simulink model "AA1111"  (R2018b)
settings: Solver=ode3  StartTime=0.0  StopTime=6000  FixedStep=T  RelTol=1e-3
PreLoadFcn:
  | Initial_LZ04
InitFcn:
  | Initial_LZ04
values from neighbouring files (symbols this model uses):
  Abg_GyroA = [0 0 1;0 1 0;-1 0 0]    [Initial_LZ04.m]
  Abg_GyroB = angle2dcm(-pi*3/4,0,-58/180*pi,'ZYX')    [Initial_LZ04.m]
  Abm_MmA = [0 -1 0;1 0 0;0 0 1]    [Initial_LZ04.m]
  Abm_MmB = [0 -1 0;1 0 0;0 0 1]    [Initial_LZ04.m]
  Att0 = 1*[80 0 0]'*pi/180    [Initial_LZ04.m]
  FixErr_StA = [15;15;15]*0*Kg_FixErr_St    [Initial_LZ04.m]
  FixErr_StB = ([15;15;15]*0+[10800;0;0])*Kg_FixErr_St    [Initial_LZ04.m]
  Fw_Mode = FW_Block(8,1)    [Initial.m]    (also in Initial_LZ04.m = 2)
  Fw_tao = 0.3    [Initial_LZ04.m]
  FwHmax = 4    [Initial_LZ04.m]
  FwTmax = FwTmax0    (= 0.05)    [Initial_LZ04.m]
  H0 = 0*[2;-2;-2;0]    [Initial_LZ04.m]
  Ib0_0 = [117.6 -1.39e-1 -1.14;-1.39e-1 101.9 -8.37e-2;-1.14 -8.37e-2 109.0]    [Initial_LZ04.m]
  jw = 0.0064    [Initial_LZ04.m]
  Matrix_I0 = [sin(50/180*pi)*cos(45/180*pi) -sin(50/180*pi)*cos(45/180*pi) -sin(50/180*pi)*cos(45/180*pi) sin(50/180*pi)*cos(45/180*pi);           sin(50/180*pi)*sin(45/180*pi) sin(50/180*pi)*sin(45/180*pi) -sin(50/180*pi)*sin(45/180*pi) -sin(50/180*pi)*sin(45/180*pi);           cos(50/180*pi) cos(50/180*pi) cos(50/180*pi) cos(50/180*pi)]    [Initial_LZ04.m]
  MtInfluence = 0    [Initial_LZ04.m]
  mu = 3.9860044e14    (= 398600440000000)    [Initial_LZ04.m]    (also in ZZ_User_Att.m)
  Ngc1 = [0.01;-0.02;-0.03]*Kg_Drift_Gyro*1+0*[0.001;-0.001;-0.001]    [Initial_LZ04.m]
  Ngc2 = [-0.02;0.01;-0.03]*Kg_Drift_Gyro    [Initial_LZ04.m]
  NgwxA = 0.005/60*sqrt(1/T_ctrl)*3*Kg_Noise_Gyro    [Initial_LZ04.m]
  NgwxB = 0.02/60*sqrt(1/T_ctrl)*3*Kg_Noise_Gyro    [Initial_LZ04.m]
  Noise_Mm = 7e-5*Kg_Noise_Mm    (= 7e-05)    [Initial_LZ04.m]
  Noise_StA = [3;3;30]*Kg_Noise_St    [Initial_LZ04.m]
  Noise_StB = [3;3;30]*Kg_Noise_St    [Initial_LZ04.m]
  OpenLoop_Att = 0    [Initial_LZ04.m]
  OpenLoop_Obt = 0    [Initial_LZ04.m]
  Qbs_StAFix = quatmultiply(angle2quat(pi,0,0,'XYZ'),angle2quat(-40/180*pi,20/180*pi,0,'XYZ'))    [Initial_LZ04.m]
  Qbs_StBFix = quatmultiply(angle2quat(pi,0,0,'XYZ'),angle2quat(40/180*pi,20/180*pi,0,'XYZ'))    [Initial_LZ04.m]
  Re = 6371.14e+3    (= 6371140)    [Initial.m]    (also in Initial_LZ04.m; ZZ_SystemApp.m)
  StartTime = [Year Month Day Hour Min Sec]'    [Initial_LZ04.m]
  T = T_PID - MainI.*[a_f/180*pi;0;0]    [Att_Ctrl.m]    (also in Initial_LZ04.m = 0.125; ZZ_Att.m = Tc(Axis))
  T_ctrl = 0.25    [Initial_LZ04.m]
  vx0 = sqrt(mu/a/(1-e^2))*(-sin(f)*sp(1)+(e+cos(f))*sq(1))    [Initial_LZ04.m]
  vy0 = sqrt(mu/a/(1-e^2))*(-sin(f)*sp(2)+(e+cos(f))*sq(2))    [Initial_LZ04.m]
  vz0 = sqrt(mu/a/(1-e^2))*(-sin(f)*sp(3)+(e+cos(f))*sq(3))    [Initial_LZ04.m]
  W_bi0 = 1*[0;-w0;0]+0*[2;-2;2]*pi/180    [Initial_LZ04.m]
  x0 = r0*(cos(omg+f)*cos(OMG)-sin(omg+f)*cos(i)*sin(OMG))    [Initial_LZ04.m]
  y0 = r0*(cos(omg+f)*sin(OMG)+sin(omg+f)*cos(i)*cos(OMG))    [Initial_LZ04.m]
  z0 = r0*sin(omg+f)*sin(i)    [Initial_LZ04.m]
undefined symbols (not defined in the file or in its folder): DiscIntNeverNeededParam, omegawXa
libraries: sharedutil x26, aerolibutil x15, simulink x12, sharedtransform x9, dspinverses x3, aerolibobsolete x1, vrlib x1
(part 3 of 3)

== system AA1111/Others/Oribit motion model/Compute osculating elements/     1/If Action Subsystem2 ==
  u : Inport
  T : Inport  Port=2
  Action Port : ActionPort  ActionType=then
  Product : Product  Inputs=3  RndMeth=Zero
  Sum : Sum  Inputs=|++  SaturateOnIntegerOverflow=on
  uz1 : Constant  Value=pi  VectorParams1D=off
  uz2 : Constant  Value=1/(2*pi)  VectorParams1D=off
  Out1 : Outport
  wires:
  u/1 -> Sum/1
  uz1/1 -> Sum/2
  Sum/1 -> Product/1
  uz2/1 -> Product/2
  Product/1 -> Out1/1
  T/1 -> Product/3

== system AA1111/Others/Oribit motion model/Compute osculating elements/   1/If Action Subsystem ==
  In1 : Inport
  Action Port : ActionPort  ActionType=then
  Out1 : Outport
  wires:
  In1/1 -> Out1/1

== system AA1111/Others/Oribit motion model/Compute osculating elements/   1/If Action Subsystem1 ==
  In1 : Inport
  Action Port : ActionPort  ActionType=else
  Constant : Constant  Value=2*pi
  Sum : Sum  Inputs=|+-  SaturateOnIntegerOverflow=on
  Out1 : Outport
  wires:
  Sum/1 -> Out1/1
  In1/1 -> Sum/2
  Constant/1 -> Sum/1

== system AA1111/Satellite Software/DataAcquisition/GyroMeasurment/TurntableModel/GyroOnTurntable ==
  dfai(¡ã/s) : Inport
  angle(¡ã) : Inport  Port=2
  Constant : Constant  Value=0
  Constant1 : Constant
  Demux1 : Demux  Outputs=3
  Gain : Gain  Gain=pi/180
  Gain1 : Gain
  Gain2 : Gain  Gain=-1
  Mux : Mux  Inputs=9
  Product : Product
  Product1 : Product
  Product2 : Product  Multiplication=Matrix(*)
  Reshape : Reshape  OutputDimensionality=Customize  OutputDimensions=[3,3]
  Terminator : Terminator
  Trigonometric Function2 : Trigonometry
  Trigonometric Function3 : Trigonometry  Operator=cos
  Trigonometric Function4 : Trigonometry
  Trigonometric Function5 : Trigonometry  Operator=cos
  wbi(¡ã/s) : Outport
  wires:
  Gain1/1 -> Mux/3
  Trigonometric Function3/1 -> Product/1, Product1/1
  Demux1/1 -> Terminator/1
  angle(¡ã)/1 -> Gain/1
  dfai(¡ã/s)/1 -> Product2/2
  Gain2/1 -> Mux/2
  Product2/1 -> wbi(¡ã/s)/1
  Reshape/1 -> Product2/1
  Constant1/1 -> Mux/9
  Product/1 -> Mux/1
  Product1/1 -> Gain2/1
  Trigonometric Function4/1 -> Product1/2, Mux/4
  Demux1/3 -> Trigonometric Function4/1, Trigonometric Function5/1
  Trigonometric Function2/1 -> Gain1/1
  Constant/1 -> Mux/6, Mux/7, Mux/8
  Mux/1 -> Reshape/1
  Gain/1 -> Demux1/1
  Trigonometric Function5/1 -> Product/2, Mux/5
  Demux1/2 -> Trigonometric Function2/1, Trigonometric Function3/1

== system AA1111/Satellite Software/DataAcquisition/GyroMeasurment/TurntableModel/Turntable Model ==
  W(¡ã/s) : Inport
  Constant : Constant  Value=360
  Demux : Demux  Outputs=3
  Integrator : Integrator
  Integrator1 : Integrator
  Integrator2 : Integrator
  Math Function : Math  Operator=mod  SaturateOnIntegerOverflow=on
  Math Function1 : Math  Operator=mod  SaturateOnIntegerOverflow=on
  Math Function2 : Math  Operator=mod  SaturateOnIntegerOverflow=on
  Mux : Mux  Inputs=3
  Angle(¡ã) : Outport
  wires:
  W(¡ã/s)/1 -> Demux/1
  Demux/1 -> Integrator/1
  Demux/2 -> Integrator1/1
  Demux/3 -> Integrator2/1
  Integrator/1 -> Math Function/1
  Mux/1 -> Angle(¡ã)/1
  Math Function/1 -> Mux/1
  Integrator1/1 -> Math Function1/1
  Integrator2/1 -> Math Function2/1
  Math Function2/1 -> Mux/3
  Math Function1/1 -> Mux/2
  Constant/1 -> Math Function2/2, Math Function1/2, Math Function/2

== system AA1111/Satellite Software/DataAcquisition/GyroMeasurment/TurntableModel/TurntableRotateSpeedCal ==
  wbi(¡ã/s) : Inport
  angle(¡ã) : Inport  Port=2
  Manual Switch : ManualSwitch
  Manual Switch1 : ManualSwitch
  TurntableRotateSpeedCal : Subsystem
  d_Att : Subsystem
  d_Att1 : Subsystem
  dfai(¡ã/s) : Outport
  wires:
  wbi(¡ã/s)/1 -> TurntableRotateSpeedCal/1(wbi(¡ã/s)), d_Att/1(wbi), d_Att1/1(wbi)
  angle(¡ã)/1 -> TurntableRotateSpeedCal/2(angle(¡ã)), d_Att/2(Att(xyz)), d_Att1/2(Att(xyz))
  TurntableRotateSpeedCal/1(dfai(¡ã/s)) -> Manual Switch/1
  d_Att/1(d_Att(xyz)) -> Manual Switch/2
  Manual Switch/1 -> Manual Switch1/1
  d_Att1/1(d_Att(xyz)) -> Manual Switch1/2
  Manual Switch1/1 -> dfai(¡ã/s)/1

== system AA1111/Satellite Software/DataAcquisition/OrbitElement measure/R//VToOrbitElement/  ==
  note: 0<=OMG<=2pi
  Hi : Inport
  Fcn1 : Fcn  Expr=u(1)
  Fcn2 : Fcn  Expr=u(2)
  If : If  IfExpression=u1 < 0
  If Action Subsystem : Subsystem  TreatAsAtomicUnit=on
  If Action Subsystem1 : Subsystem  TreatAsAtomicUnit=on
  Merge : Merge
  Mux3 : Mux  Inputs=2
  tg(OMG)=Hxi/(-Hyi) : Fcn  Expr=atan2(u[1],-u[2])
  OMG : Outport
  wires:
  Fcn1/1 -> Mux3/1
  Fcn2/1 -> Mux3/2
  Mux3/1 -> tg(OMG)=Hxi/(-Hyi)/1
  tg(OMG)=Hxi/(-Hyi)/1 -> If/1, If Action Subsystem/1(In1), If Action Subsystem1/1(In1)
  If/1 -> If Action Subsystem/Action
  If/2 -> If Action Subsystem1/Action
  If Action Subsystem/1(Out1) -> Merge/1
  If Action Subsystem1/1(Out1) -> Merge/2
  Merge/1 -> OMG/1
  Hi/1 -> Fcn1/1, Fcn2/1

== system AA1111/Satellite Software/DataAcquisition/OrbitElement measure/R//VToOrbitElement/      ==
  H_xyz : Inport
  R_xyz : Inport  Port=2
  3x3 Cross Product : sharedutil/3x3 Cross Product  aMode=aMode
      settings: SourceProductBaseCode=AE
  Dot Product4 : DotProduct  InputSameDT=on  OutDataTypeStr=Inherit: Inherit via internal rule
  Fcn1 : Fcn  Expr=acos(u[2]/(u[1]*u[3]))
  Fcn3 : Fcn  Expr=sqrt(u[1]^2+u[2]^2+u[3]^2)
  Fcn4 : Fcn  Expr=u[3]
  Fcn5 : Fcn  Expr=sqrt(u[1]^2+u[2]^2+u[3]^2)
  If Action Subsystem2 : Subsystem  TreatAsAtomicUnit=on
  If Action Subsystem3 : Subsystem  TreatAsAtomicUnit=on
  If1 : If
  Merge1 : Merge
  Mux1 : Mux  Inputs=3
  uz : Constant  Value=[0;0;1]  VectorParams1D=off
  u : Outport
  wires:
  uz/1 -> 3x3 Cross Product/1
  H_xyz/1 -> 3x3 Cross Product/2
  3x3 Cross Product/1 -> Dot Product4/1, Fcn5/1
  R_xyz/1 -> Fcn3/1, Dot Product4/2, Fcn4/1
  Fcn3/1 -> Mux1/3
  Dot Product4/1 -> Mux1/2
  Mux1/1 -> Fcn1/1
  Fcn4/1 -> If1/1
  If1/1 -> If Action Subsystem2/Action
  Fcn1/1 -> If Action Subsystem2/1(In1), If Action Subsystem3/1(In1)
  If Action Subsystem2/1(Out1) -> Merge1/1
  If Action Subsystem3/1(Out1) -> Merge1/2
  Merge1/1 -> u/1
  Fcn5/1 -> Mux1/1
  If1/2 -> If Action Subsystem3/Action

== system AA1111/Satellite Software/DataAcquisition/OrbitElement measure/R//VToOrbitElement/     1 ==
  note: Orbit Period T
  u : Inport
  a : Inport  Port=2
  Fcn : Fcn  Expr=2*pi*sqrt(u(1)^3/mu)
  If Action Subsystem1 : Subsystem  TreatAsAtomicUnit=on
  If Action Subsystem2 : Subsystem  TreatAsAtomicUnit=on
  If1 : If  IfExpression=u1 <pi
  Merge1 : Merge
  OrbitClock : Outport
  wires:
  If1/2 -> If Action Subsystem1/Action
  Merge1/1 -> OrbitClock/1
  If Action Subsystem1/1(Out1) -> Merge1/2
  If Action Subsystem2/1(Out1) -> Merge1/1
  If1/1 -> If Action Subsystem2/Action
  u/1 -> If Action Subsystem2/1(u), If1/1, If Action Subsystem1/1(u)
  a/1 -> Fcn/1
  Fcn/1 -> If Action Subsystem2/2(T), If Action Subsystem1/2(T)

== system AA1111/Satellite Software/DataAcquisition/OrbitElement measure/R//VToOrbitElement/   1 ==
  note: 0<=omg<=2pi
  note: Éý½»µãÊ¸Á¿Óë½üµØµãÊ¸Á¿µÄ¼Ð½Ç
  note: ¹ìµÀ½ÚÏßÊ¸Á¿N
  H_xyz : Inport
  V_xyz : Inport  Port=2
  R_xyz : Inport  Port=3
  3x3 Cross Product : sharedutil/3x3 Cross Product  aMode=aMode
      settings: SourceProductBaseCode=AE
  3x3 Cross Product1 : sharedutil/3x3 Cross Product  aMode=aMode
      settings: SourceProductBaseCode=AE
  Divide : Product  Inputs=*/
  Dot Product3 : DotProduct  InputSameDT=on  OutDataTypeStr=Inherit: Inherit via internal rule
  Fcn : Fcn  Expr=acos(u[2]/(u[1]*u[3]))
  Fcn2 : Fcn  Expr=u[3]
  Fcn3 : Fcn  Expr=sqrt(u[1]^2+u[2]^2+u[3]^2)
  Fcn5 : Fcn  Expr=sqrt(u[1]^2+u[2]^2+u[3]^2)
  Fcn6 : Fcn  Expr=sqrt(u[1]^2+u[2]^2+u[3]^2)
  Gain1 : Gain  Gain=180/pi
  Gain3 : Gain  Gain=mu  SaturateOnIntegerOverflow=on  OutDataTypeStr=Inherit: Same as input  ParamDataTypeStr=Inherit: Same as input
  If : If  IfExpression=u1 >= 0
  If Action Subsystem : Subsystem  TreatAsAtomicUnit=on
  If Action Subsystem1 : Subsystem  TreatAsAtomicUnit=on
  Merge : Merge
  Mux : Mux  Inputs=3
  Sum : Sum  Inputs=|--  SaturateOnIntegerOverflow=on
  uz : Constant  Value=[0;0;1]  VectorParams1D=off
  w{,1..4} (5 alike) : Scope
  omg : Outport
  wires:
  H_xyz/1 -> 3x3 Cross Product/2, 3x3 Cross Product1/1
  If Action Subsystem1/1(Out1) -> Merge/2
  If Action Subsystem/1(Out1) -> Merge/1
  Fcn/1 -> If Action Subsystem1/1(In1), If Action Subsystem/1(In1), Gain1/1
  Fcn2/1 -> If/1, w1/1
  Mux/1 -> Fcn/1
  Fcn6/1 -> Mux/3, w4/1
  Sum/1 -> Fcn2/1, Dot Product3/2, Fcn6/1
  Divide/1 -> Sum/2, w2/1
  Fcn3/1 -> Divide/2
  3x3 Cross Product/1 -> Fcn5/1, Dot Product3/1
  uz/1 -> 3x3 Cross Product/1
  3x3 Cross Product1/1 -> Sum/1, w3/1
  R_xyz/1 -> Fcn3/1, Gain3/1
  Dot Product3/1 -> Mux/2
  V_xyz/1 -> 3x3 Cross Product1/2
  Merge/1 -> omg/1
  If/1 -> If Action Subsystem/Action
  If/2 -> If Action Subsystem1/Action
  Gain1/1 -> w/1
  Gain3/1 -> Divide/1
  Fcn5/1 -> Mux/1

== system AA1111/Satellite Software/DataAcquisition/OrbitElement measure/qip/2 ==
  q : Inport
  Demux : Demux
  Gain1 : Gain  Gain=-1  SaturateOnIntegerOverflow=on  OutDataTypeStr=Inherit: Same as input  ParamDataTypeStr=Inherit: Same as input
  Gain2 : Gain  Gain=-1  SaturateOnIntegerOverflow=on  OutDataTypeStr=Inherit: Same as input  ParamDataTypeStr=Inherit: Same as input
  Gain3 : Gain  Gain=-1  SaturateOnIntegerOverflow=on  OutDataTypeStr=Inherit: Same as input  ParamDataTypeStr=Inherit: Same as input
  Mux : Mux
  inv(q) : Outport
  wires:
  Gain3/1 -> Mux/4
  Demux/4 -> Gain3/1
  Demux/3 -> Gain2/1
  Demux/2 -> Gain1/1
  Demux/1 -> Mux/1
  Gain2/1 -> Mux/3
  Gain1/1 -> Mux/2
  Mux/1 -> inv(q)/1
  q/1 -> Demux/1

== system AA1111/Others/Attitude Kinematics Equations & Attitude Dynamics Equations/Kinetics/Qob 2 Qib/qip/2 ==
  q : Inport
  Demux : Demux
  Gain1 : Gain  Gain=-1  SaturateOnIntegerOverflow=on  OutDataTypeStr=Inherit: Same as input  ParamDataTypeStr=Inherit: Same as input
  Gain2 : Gain  Gain=-1  SaturateOnIntegerOverflow=on  OutDataTypeStr=Inherit: Same as input  ParamDataTypeStr=Inherit: Same as input
  Gain3 : Gain  Gain=-1  SaturateOnIntegerOverflow=on  OutDataTypeStr=Inherit: Same as input  ParamDataTypeStr=Inherit: Same as input
  Mux : Mux
  inv(q) : Outport
  wires:
  q/1 -> Demux/1
  Mux/1 -> inv(q)/1
  Gain1/1 -> Mux/2
  Gain2/1 -> Mux/3
  Demux/1 -> Mux/1
  Demux/2 -> Gain1/1
  Demux/3 -> Gain2/1
  Demux/4 -> Gain3/1
  Gain3/1 -> Mux/4

== system AA1111/Others/Attitude Kinematics Equations & Attitude Dynamics Equations/Kinetics/Qob 2 Qib1/qip/2 ==
  q : Inport
  Demux : Demux
  Gain1 : Gain  Gain=-1  SaturateOnIntegerOverflow=on  OutDataTypeStr=Inherit: Same as input  ParamDataTypeStr=Inherit: Same as input
  Gain2 : Gain  Gain=-1  SaturateOnIntegerOverflow=on  OutDataTypeStr=Inherit: Same as input  ParamDataTypeStr=Inherit: Same as input
  Gain3 : Gain  Gain=-1  SaturateOnIntegerOverflow=on  OutDataTypeStr=Inherit: Same as input  ParamDataTypeStr=Inherit: Same as input
  Mux : Mux
  inv(q) : Outport
  wires:
  Gain3/1 -> Mux/4
  Demux/4 -> Gain3/1
  Demux/3 -> Gain2/1
  Demux/2 -> Gain1/1
  Demux/1 -> Mux/1
  Gain2/1 -> Mux/3
  Gain1/1 -> Mux/2
  Mux/1 -> inv(q)/1
  q/1 -> Demux/1

== system AA1111/Others/Disturbing torque/Compute geomagnetism1/Subsystem/Subsystem1/-pi~pi ==
  In1 : Inport
  If Action Subsystem1 : Subsystem  TreatAsAtomicUnit=on
  If Action Subsystem2 : Subsystem  TreatAsAtomicUnit=on
  If Action Subsystem3 : Subsystem  TreatAsAtomicUnit=on
  If Action Subsystem4 : Subsystem  TreatAsAtomicUnit=on
  If1 : If  IfExpression=u1>pi
  If2 : If  IfExpression=u1<0
  Merge1 : Merge
  Merge2 : Merge
  Out1 : Outport
  wires:
  Merge2/1 -> If Action Subsystem3/1(In), If Action Subsystem4/1(In), If1/1
  If Action Subsystem2/1(Out) -> Merge2/2
  If Action Subsystem1/1(Out) -> Merge2/1
  If2/2 -> If Action Subsystem2/Action
  If2/1 -> If Action Subsystem1/Action
  In1/1 -> If Action Subsystem2/1(In), If Action Subsystem1/1(In), If2/1
  Merge1/1 -> Out1/1
  If1/1 -> If Action Subsystem4/Action
  If Action Subsystem4/1(Out) -> Merge1/1
  If1/2 -> If Action Subsystem3/Action
  If Action Subsystem3/1(Out) -> Merge1/2

== system AA1111/Others/Disturbing torque/Compute geomagnetism1/Subsystem/Subsystem1/-pi~pi1 ==
  In1 : Inport
  If Action Subsystem1 : Subsystem  TreatAsAtomicUnit=on
  If Action Subsystem2 : Subsystem  TreatAsAtomicUnit=on
  If Action Subsystem3 : Subsystem  TreatAsAtomicUnit=on
  If Action Subsystem4 : Subsystem  TreatAsAtomicUnit=on
  If1 : If  IfExpression=u1>pi
  If2 : If  IfExpression=u1<0
  Merge1 : Merge
  Merge2 : Merge
  Out1 : Outport
  wires:
  If Action Subsystem3/1(Out) -> Merge1/2
  If1/2 -> If Action Subsystem3/Action
  If Action Subsystem4/1(Out) -> Merge1/1
  If1/1 -> If Action Subsystem4/Action
  Merge1/1 -> Out1/1
  In1/1 -> If2/1, If Action Subsystem1/1(In), If Action Subsystem2/1(In)
  If2/1 -> If Action Subsystem1/Action
  If2/2 -> If Action Subsystem2/Action
  If Action Subsystem1/1(Out) -> Merge2/1
  If Action Subsystem2/1(Out) -> Merge2/2
  Merge2/1 -> If1/1, If Action Subsystem4/1(In), If Action Subsystem3/1(In)

== system AA1111/Others/Disturbing torque/Compute geomagnetism1/Subsystem/Subsystem1/If Action Subsystem1 ==
  In : Inport
  Action Port : ActionPort  ActionType=else
  Demux : Demux  Outputs=2
  If : If  NumInputs=2  IfExpression=u2>0
  If Action Subsystem1 : Subsystem  TreatAsAtomicUnit=on
  If Action Subsystem2 : Subsystem  TreatAsAtomicUnit=on
  Merge : Merge
  Out : Outport
  wires:
  If/1 -> If Action Subsystem1/Action
  In/1 -> Demux/1
  Demux/1 -> If/1
  Demux/2 -> If/2
  If/2 -> If Action Subsystem2/Action
  If Action Subsystem1/1(Out) -> Merge/1
  If Action Subsystem2/1(Out) -> Merge/2
  Merge/1 -> Out/1

== system AA1111/Others/Disturbing torque/Compute geomagnetism1/Subsystem/Subsystem1/If Action Subsystem2 ==
  In : Inport
  Action Port : ActionPort  ActionType=then
  Fcn4 : Fcn  Expr=atan2(u[2],u[1])
  Out : Outport
  wires:
  In/1 -> Fcn4/1
  Fcn4/1 -> Out/1

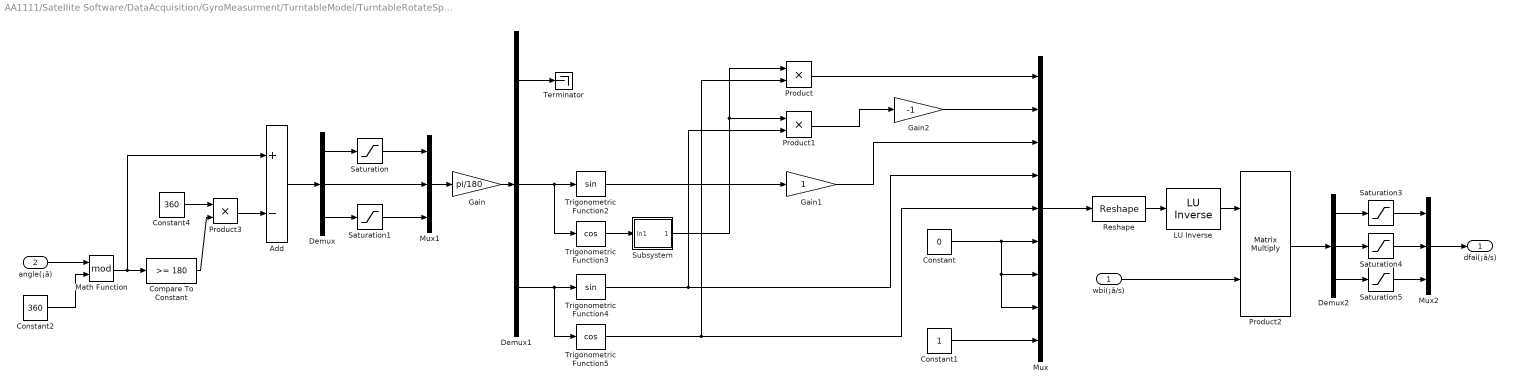
== system AA1111/Satellite Software/DataAcquisition/GyroMeasurment/TurntableModel/TurntableRotateSpeedCal/TurntableRotateSpeedCal ==
  wbi(¡ã/s) : Inport
  angle(¡ã) : Inport  Port=2
  " LU Inverse" : dspinverses/ LU Inverse
      settings: SourceProductName=DSP System Toolbox
  Add : Sum  Inputs=+-
  Compare To Constant : simulink/Logic and Bit Operations/Compare To Constant  relop=>=  const=180  OutDataTypeStr=uint8
  Constant : Constant  Value=0
  Constant1 : Constant
  Constant2 : Constant  Value=360
  Constant4 : Constant  Value=360
  Demux : Demux  Outputs=3
  Demux1 : Demux  Outputs=3
  Demux2 : Demux  Outputs=3
  Gain : Gain  Gain=pi/180
  Gain1 : Gain
  Gain2 : Gain  Gain=-1
  Math Function : Math  Operator=mod  SaturateOnIntegerOverflow=on
  Mux : Mux  Inputs=9
  Mux1 : Mux  Inputs=3
  Mux2 : Mux  Inputs=3
  Product : Product
  Product1 : Product
  Product2 : Product  Multiplication=Matrix(*)
  Product3 : Product
  Reshape : Reshape  OutputDimensionality=Customize  OutputDimensions=[3,3]
  Saturation : Saturate  UpperLimit=179  LowerLimit=-179
  Saturation1 : Saturate  UpperLimit=179  LowerLimit=-179
  Saturation3 : Saturate  UpperLimit=5  LowerLimit=-5
  Saturation4 : Saturate  UpperLimit=5  LowerLimit=-5
  Saturation5 : Saturate  UpperLimit=5  LowerLimit=-5
  Subsystem : Subsystem
  Terminator : Terminator
  Trigonometric Function2 : Trigonometry
  Trigonometric Function3 : Trigonometry  Operator=cos
  Trigonometric Function4 : Trigonometry
  Trigonometric Function5 : Trigonometry  Operator=cos
  dfai(¡ã/s) : Outport
  wires:
  Demux1/2 -> Trigonometric Function3/1, Trigonometric Function2/1
  Trigonometric Function5/1 -> Mux/5, Product/2
  Gain/1 -> Demux1/1
  Mux/1 -> Reshape/1
  Constant/1 -> Mux/6, Mux/7, Mux/8
  Trigonometric Function2/1 -> Gain1/1
  Demux1/3 -> Trigonometric Function5/1, Trigonometric Function4/1
  Trigonometric Function4/1 -> Product1/2, Mux/4
  Product1/1 -> Gain2/1
  Product/1 -> Mux/1
  Constant1/1 -> Mux/9
  " LU Inverse"/1 -> Product2/1
  Reshape/1 -> " LU Inverse"/1
  Math Function/1 -> Add/1, Compare To Constant/1
  Constant2/1 -> Math Function/2
  Constant4/1 -> Product3/1
  Compare To Constant/1 -> Product3/2
  Product3/1 -> Add/2
  Add/1 -> Demux/1
  Gain2/1 -> Mux/2
  Demux/2 -> Mux1/2
  Demux/3 -> Saturation1/1
  Saturation/1 -> Mux1/1
  Mux1/1 -> Gain/1
  Demux/1 -> Saturation/1
  Saturation1/1 -> Mux1/3
  wbi(¡ã/s)/1 -> Product2/2
  angle(¡ã)/1 -> Math Function/1
  Demux1/1 -> Terminator/1
  Subsystem/1(Out1) -> Product1/1, Product/1
  Trigonometric Function3/1 -> Subsystem/1(In1)
  Gain1/1 -> Mux/3
  Demux2/2 -> Saturation4/1
  Demux2/3 -> Saturation5/1
  Saturation3/1 -> Mux2/1
  Mux2/1 -> dfai(¡ã/s)/1
  Demux2/1 -> Saturation3/1
  Saturation5/1 -> Mux2/3
  Saturation4/1 -> Mux2/2
  Product2/1 -> Demux2/1

== system AA1111/Satellite Software/DataAcquisition/GyroMeasurment/TurntableModel/TurntableRotateSpeedCal/d_Att ==
  note: 0.0349 ¶ÔÓ¦88deg
      | 0.0872¶ÔÓ¦85deg
  wbi : Inport
  Att(xyz) : Inport  Port=2
  Demux2 : Demux  Outputs=3
  Fcn : Fcn  Expr=abs(cos(u(2)/180*pi))
  If : If  IfExpression=u1 <= 0.0349
  If Action Subsystem1 : Subsystem  TreatAsAtomicUnit=on
  If Action Subsystem2 : Subsystem  TreatAsAtomicUnit=on
  Integer Delay : Delay  DelayLength=1  InputProcessing=Inherited
  Merge : Merge
  Mux2 : Mux  Inputs=3
  Saturation3 : Saturate  UpperLimit=5  LowerLimit=-5
  Saturation4 : Saturate  UpperLimit=5  LowerLimit=-5
  Saturation5 : Saturate  UpperLimit=5  LowerLimit=-5
  d_Att(xyz) : Outport
  wires:
  If Action Subsystem2/1(Out2) -> Merge/1
  If/1 -> If Action Subsystem2/Action
  If Action Subsystem1/1(dfai(¡ã/s)) -> Merge/2
  If/2 -> If Action Subsystem1/Action
  Fcn/1 -> If/1
  Att(xyz)/1 -> If Action Subsystem1/2(angle(¡ã)), Fcn/1
  wbi/1 -> If Action Subsystem1/1(wbi(¡ã/s))
  Integer Delay/1 -> If Action Subsystem2/1(In2)
  Demux2/2 -> Saturation4/1
  Demux2/3 -> Saturation5/1
  Saturation3/1 -> Mux2/1
  Mux2/1 -> d_Att(xyz)/1, Integer Delay/1
  Demux2/1 -> Saturation3/1
  Saturation5/1 -> Mux2/3
  Saturation4/1 -> Mux2/2
  Merge/1 -> Demux2/1

== system AA1111/Satellite Software/DataAcquisition/GyroMeasurment/TurntableModel/TurntableRotateSpeedCal/d_Att1 ==
  wbi : Inport
  Att(xyz) : Inport  Port=2
  Demux2 : Demux  Outputs=3
  If Action Subsystem1 : Subsystem  TreatAsAtomicUnit=on
  Mux2 : Mux  Inputs=3
  Saturation3 : Saturate  UpperLimit=5  LowerLimit=-5
  Saturation4 : Saturate  UpperLimit=5  LowerLimit=-5
  Saturation5 : Saturate  UpperLimit=5  LowerLimit=-5
  d_Att(xyz) : Outport
  wires:
  Saturation4/1 -> Mux2/2
  Saturation5/1 -> Mux2/3
  Demux2/1 -> Saturation3/1
  Mux2/1 -> d_Att(xyz)/1
  Saturation3/1 -> Mux2/1
  Demux2/3 -> Saturation5/1
  Demux2/2 -> Saturation4/1
  wbi/1 -> If Action Subsystem1/1(wbi(¡ã/s))
  Att(xyz)/1 -> If Action Subsystem1/2(angle(¡ã))
  If Action Subsystem1/1(dfai(¡ã/s)) -> Demux2/1

== system AA1111/Satellite Software/DataAcquisition/OrbitElement measure/R//VToOrbitElement/ /If Action Subsystem ==
  note: In+2pi, due to OMG's Range=[0 2*pi],
      | and atan2's Range=[-pi pi]
  In1 : Inport
  Action Port : ActionPort  ActionType=then
  Constant : Constant  Value=2*pi
  Sum : Sum  Inputs=|++  SaturateOnIntegerOverflow=on
  Out1 : Outport
  wires:
  In1/1 -> Sum/1
  Sum/1 -> Out1/1
  Constant/1 -> Sum/2

== system AA1111/Satellite Software/DataAcquisition/OrbitElement measure/R//VToOrbitElement/ /If Action Subsystem1 ==
  In1 : Inport
  Action Port : ActionPort  ActionType=else
  Out1 : Outport
  wires:
  In1/1 -> Out1/1

== system AA1111/Satellite Software/DataAcquisition/OrbitElement measure/R//VToOrbitElement/     /If Action Subsystem2 ==
  In1 : Inport
  Action Port : ActionPort  ActionType=then
  Out1 : Outport
  wires:
  In1/1 -> Out1/1

== system AA1111/Satellite Software/DataAcquisition/OrbitElement measure/R//VToOrbitElement/     /If Action Subsystem3 ==
  In1 : Inport
  Action Port : ActionPort  ActionType=else
  Constant : Constant  Value=2*pi
  Sum : Sum  Inputs=|+-  SaturateOnIntegerOverflow=on
  Out1 : Outport
  wires:
  Sum/1 -> Out1/1
  In1/1 -> Sum/2
  Constant/1 -> Sum/1

== system AA1111/Satellite Software/DataAcquisition/OrbitElement measure/R//VToOrbitElement/     1/If Action Subsystem1 ==
  u : Inport
  T : Inport  Port=2
  Action Port : ActionPort  ActionType=else
  Product : Product  Inputs=3  RndMeth=Zero
  Sum : Sum  Inputs=|+-  SaturateOnIntegerOverflow=on
  uz1 : Constant  Value=pi  VectorParams1D=off
  uz2 : Constant  Value=1/(2*pi)  VectorParams1D=off
  Out1 : Outport
  wires:
  Product/1 -> Out1/1
  uz2/1 -> Product/2
  Sum/1 -> Product/1
  uz1/1 -> Sum/2
  u/1 -> Sum/1
  T/1 -> Product/3

== system AA1111/Satellite Software/DataAcquisition/OrbitElement measure/R//VToOrbitElement/     1/If Action Subsystem2 ==
  u : Inport
  T : Inport  Port=2
  Action Port : ActionPort  ActionType=then
  Product : Product  Inputs=3  RndMeth=Zero
  Sum : Sum  Inputs=|++  SaturateOnIntegerOverflow=on
  uz1 : Constant  Value=pi  VectorParams1D=off
  uz2 : Constant  Value=1/(2*pi)  VectorParams1D=off
  Out1 : Outport
  wires:
  u/1 -> Sum/1
  uz1/1 -> Sum/2
  Sum/1 -> Product/1
  uz2/1 -> Product/2
  Product/1 -> Out1/1
  T/1 -> Product/3

== system AA1111/Satellite Software/DataAcquisition/OrbitElement measure/R//VToOrbitElement/   1/If Action Subsystem ==
  In1 : Inport
  Action Port : ActionPort  ActionType=then
  Out1 : Outport
  wires:
  In1/1 -> Out1/1

== system AA1111/Satellite Software/DataAcquisition/OrbitElement measure/R//VToOrbitElement/   1/If Action Subsystem1 ==
  In1 : Inport
  Action Port : ActionPort  ActionType=else
  Constant : Constant  Value=2*pi
  Sum : Sum  Inputs=|+-  SaturateOnIntegerOverflow=on
  Out1 : Outport
  wires:
  Sum/1 -> Out1/1
  In1/1 -> Sum/2
  Constant/1 -> Sum/1

== system AA1111/Others/Disturbing torque/Compute geomagnetism1/Subsystem/Subsystem1/-pi~pi/If Action Subsystem1 ==
  In : Inport
  Action Port : ActionPort  ActionType=then
  Fcn4 : Fcn  Expr=u(1)+2*pi
  Out : Outport
  wires:
  In/1 -> Fcn4/1
  Fcn4/1 -> Out/1

== system AA1111/Others/Disturbing torque/Compute geomagnetism1/Subsystem/Subsystem1/-pi~pi/If Action Subsystem2 ==
  In : Inport
  Action Port : ActionPort  ActionType=else
  Out : Outport
  wires:
  In/1 -> Out/1

== system AA1111/Others/Disturbing torque/Compute geomagnetism1/Subsystem/Subsystem1/-pi~pi/If Action Subsystem3 ==
  In : Inport
  Action Port : ActionPort  ActionType=else
  Out : Outport
  wires:
  In/1 -> Out/1

== system AA1111/Others/Disturbing torque/Compute geomagnetism1/Subsystem/Subsystem1/-pi~pi/If Action Subsystem4 ==
  In : Inport
  Action Port : ActionPort  ActionType=then
  Fcn4 : Fcn  Expr=u(1)-2*pi
  Out : Outport
  wires:
  Fcn4/1 -> Out/1
  In/1 -> Fcn4/1

== system AA1111/Others/Disturbing torque/Compute geomagnetism1/Subsystem/Subsystem1/-pi~pi1/If Action Subsystem1 ==
  In : Inport
  Action Port : ActionPort  ActionType=then
  Fcn4 : Fcn  Expr=u(1)+2*pi
  Out : Outport
  wires:
  Fcn4/1 -> Out/1
  In/1 -> Fcn4/1

== system AA1111/Others/Disturbing torque/Compute geomagnetism1/Subsystem/Subsystem1/-pi~pi1/If Action Subsystem2 ==
  In : Inport
  Action Port : ActionPort  ActionType=else
  Out : Outport
  wires:
  In/1 -> Out/1

== system AA1111/Others/Disturbing torque/Compute geomagnetism1/Subsystem/Subsystem1/-pi~pi1/If Action Subsystem3 ==
  In : Inport
  Action Port : ActionPort  ActionType=else
  Out : Outport
  wires:
  In/1 -> Out/1

== system AA1111/Others/Disturbing torque/Compute geomagnetism1/Subsystem/Subsystem1/-pi~pi1/If Action Subsystem4 ==
  In : Inport
  Action Port : ActionPort  ActionType=then
  Fcn4 : Fcn  Expr=u(1)-2*pi
  Out : Outport
  wires:
  In/1 -> Fcn4/1
  Fcn4/1 -> Out/1

== system AA1111/Others/Disturbing torque/Compute geomagnetism1/Subsystem/Subsystem1/If Action Subsystem1/If Action Subsystem1 ==
  Action Port : ActionPort  ActionType=then
  Constant : Constant  Value=pi/2
  Out : Outport  InitialOutput=pi/2
  wires:
  Constant/1 -> Out/1

== system AA1111/Others/Disturbing torque/Compute geomagnetism1/Subsystem/Subsystem1/If Action Subsystem1/If Action Subsystem2 ==
  Action Port : ActionPort  ActionType=else
  Constant : Constant  Value=3*pi/2
  Out : Outport  InitialOutput=1.5*pi
  wires:
  Constant/1 -> Out/1

== system AA1111/Satellite Software/DataAcquisition/GyroMeasurment/TurntableModel/TurntableRotateSpeedCal/TurntableRotateSpeedCal/Subsystem ==
  In1 : Inport
  Abs1 : Abs
  Constant1 : Constant  Value=0.005
  Product1 : Product
  Sign : Signum
  Switch : Switch  Criteria=u2 > Threshold  Threshold=0.005
  Out1 : Outport
  wires:
  Abs1/1 -> Switch/2
  Sign/1 -> Product1/1
  Constant1/1 -> Product1/2
  Product1/1 -> Switch/3
  Switch/1 -> Out1/1
  In1/1 -> Switch/1, Abs1/1, Sign/1

== system AA1111/Satellite Software/DataAcquisition/GyroMeasurment/TurntableModel/TurntableRotateSpeedCal/d_Att/If Action Subsystem1 ==
  wbi(¡ã/s) : Inport
  angle(¡ã) : Inport  Port=2
  Action Port : ActionPort  ActionType=else
  " LU Inverse" : dspinverses/ LU Inverse
      settings: SourceProductName=DSP System Toolbox
  Constant : Constant  Value=0
  Constant1 : Constant
  Demux1 : Demux  Outputs=3
  Gain : Gain  Gain=pi/180
  Gain1 : Gain
  Gain2 : Gain  Gain=-1
  Mux : Mux  Inputs=9
  Product : Product
  Product1 : Product
  Product2 : Product  Multiplication=Matrix(*)
  Reshape : Reshape  OutputDimensionality=Customize  OutputDimensions=[3,3]
  Terminator : Terminator
  Trigonometric Function2 : Trigonometry
  Trigonometric Function3 : Trigonometry  Operator=cos
  Trigonometric Function4 : Trigonometry
  Trigonometric Function5 : Trigonometry  Operator=cos
  dfai(¡ã/s) : Outport
  wires:
  Gain1/1 -> Mux/3
  Trigonometric Function3/1 -> Product/1, Product1/1
  Demux1/1 -> Terminator/1
  angle(¡ã)/1 -> Gain/1
  wbi(¡ã/s)/1 -> Product2/2
  Gain2/1 -> Mux/2
  Product2/1 -> dfai(¡ã/s)/1
  Reshape/1 -> " LU Inverse"/1
  " LU Inverse"/1 -> Product2/1
  Constant1/1 -> Mux/9
  Product/1 -> Mux/1
  Product1/1 -> Gain2/1
  Trigonometric Function4/1 -> Product1/2, Mux/4
  Demux1/3 -> Trigonometric Function4/1, Trigonometric Function5/1
  Trigonometric Function2/1 -> Gain1/1
  Constant/1 -> Mux/6, Mux/7, Mux/8
  Mux/1 -> Reshape/1
  Gain/1 -> Demux1/1
  Trigonometric Function5/1 -> Product/2, Mux/5
  Demux1/2 -> Trigonometric Function2/1, Trigonometric Function3/1

== system AA1111/Satellite Software/DataAcquisition/GyroMeasurment/TurntableModel/TurntableRotateSpeedCal/d_Att/If Action Subsystem2 ==
  In2 : Inport
  Action Port : ActionPort  ActionType=then
  Out2 : Outport
  wires:
  In2/1 -> Out2/1

== system AA1111/Satellite Software/DataAcquisition/GyroMeasurment/TurntableModel/TurntableRotateSpeedCal/d_Att1/If Action Subsystem1 ==
  wbi(¡ã/s) : Inport
  angle(¡ã) : Inport  Port=2
  " LU Inverse" : dspinverses/ LU Inverse
      settings: SourceProductName=DSP System Toolbox
  Constant : Constant  Value=0
  Constant1 : Constant
  Demux1 : Demux  Outputs=3
  Gain : Gain  Gain=pi/180
  Gain1 : Gain
  Gain2 : Gain  Gain=-1
  Mux : Mux  Inputs=9
  Product : Product
  Product1 : Product
  Product2 : Product  Multiplication=Matrix(*)
  Reshape : Reshape  OutputDimensionality=Customize  OutputDimensions=[3,3]
  Terminator : Terminator
  Trigonometric Function2 : Trigonometry
  Trigonometric Function3 : Trigonometry  Operator=cos
  Trigonometric Function4 : Trigonometry
  Trigonometric Function5 : Trigonometry  Operator=cos
  dfai(¡ã/s) : Outport
  wires:
  Demux1/2 -> Trigonometric Function3/1, Trigonometric Function2/1
  Trigonometric Function5/1 -> Mux/5, Product/2
  Gain/1 -> Demux1/1
  Mux/1 -> Reshape/1
  Constant/1 -> Mux/8, Mux/7, Mux/6
  Trigonometric Function2/1 -> Gain1/1
  Demux1/3 -> Trigonometric Function5/1, Trigonometric Function4/1
  Trigonometric Function4/1 -> Mux/4, Product1/2
  Product1/1 -> Gain2/1
  Product/1 -> Mux/1
  Constant1/1 -> Mux/9
  " LU Inverse"/1 -> Product2/1
  Reshape/1 -> " LU Inverse"/1
  Product2/1 -> dfai(¡ã/s)/1
  Gain2/1 -> Mux/2
  wbi(¡ã/s)/1 -> Product2/2
  angle(¡ã)/1 -> Gain/1
  Demux1/1 -> Terminator/1
  Trigonometric Function3/1 -> Product1/1, Product/1
  Gain1/1 -> Mux/3
